simulink model "lab7_sin_triangle_generator_inverter"  (R2024b)
settings: Solver=VariableStepAuto  StartTime=0.0  StopTime=1  RelTol=1e-3
libraries: spsIdealSwitchLib x4, spsTriangleGeneratorLib x2, spsDCVoltageSourceLib x1, spsSeriesRLCBranchLib x1, spsVoltageMeasurementLib x1, sps_lib x1
settings Model: Creator=Admin  LastModifiedBy=pragy
settings DataIOCC: ReturnWorkspaceOutputs=off

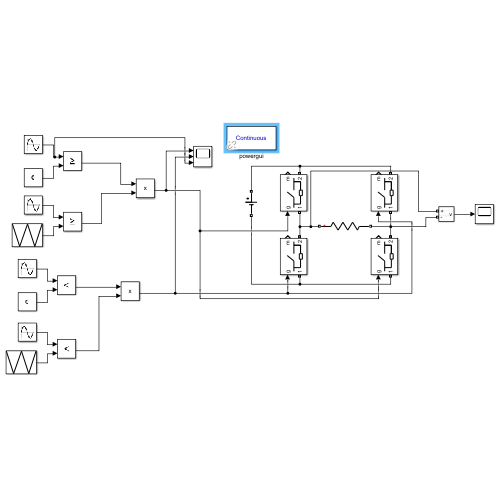
[thumbnail: Simulink's stored preview of the top-level diagram]
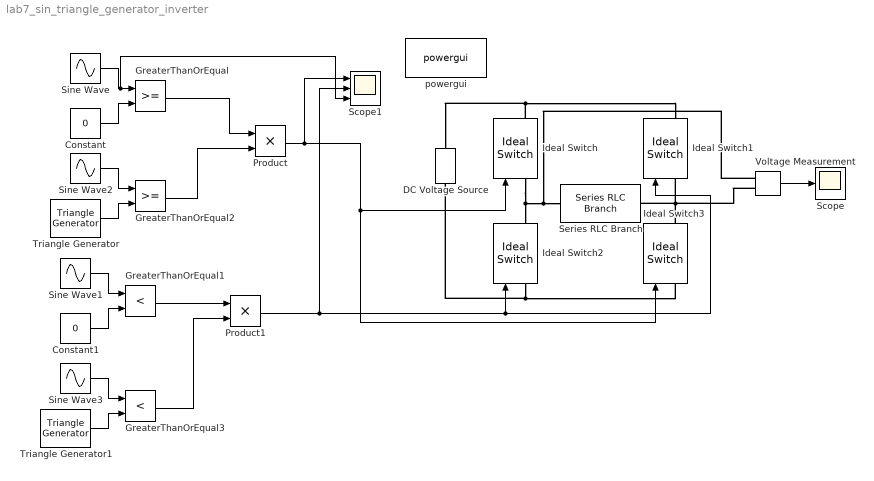
== system lab7_sin_triangle_generator_inverter ==
  Constant : Constant  Value=0
  Constant1 : Constant  Value=0
  DC Voltage Source : spsDCVoltageSourceLib/DC Voltage Source  Amplitude=220  Measurements=None
  GreaterThanOrEqual : RelationalOperator  OutDataTypeStr=boolean  RndMeth=Simplest  InputSameDT=off
  GreaterThanOrEqual1 : RelationalOperator  Operator=<  OutDataTypeStr=boolean  RndMeth=Simplest  InputSameDT=off
  GreaterThanOrEqual2 : RelationalOperator  OutDataTypeStr=boolean  RndMeth=Simplest  InputSameDT=off
  GreaterThanOrEqual3 : RelationalOperator  Operator=<  OutDataTypeStr=boolean  RndMeth=Simplest  InputSameDT=off
  Ideal Switch{,1..3} (4 alike) : spsIdealSwitchLib/Ideal Switch  Ron=0.001  Lon=0  IC=0  Rs=1e5  Cs=inf  Measurements=on
  Product : Product
  Product1 : Product
  Scope : Scope
  Scope1 : Scope  NumInputPorts=3
  Series RLC Branch : spsSeriesRLCBranchLib/Series RLC Branch  LConnTagsString=__new0  RConnTagsString=__new0  BranchType=R  Resistance=10  Inductance=1e-3  SetiL0=off  InitialCurrent=0  Capacitance=1e-6  Setx0=off  InitialVoltage=0  Measurements=None
  Sine Wave{,1..3} (4 alike) : Sin  Frequency=2*pi*50  SampleTime=0
  Triangle Generator : spsTriangleGeneratorLib/Triangle Generator  Freq=1050  Phase=180  Ts=0
  Triangle Generator1 : spsTriangleGeneratorLib/Triangle Generator  Freq=1050  Phase=180  Ts=0
  Voltage Measurement : spsVoltageMeasurementLib/Voltage Measurement  PhasorSimulation=off  OutputType=Complex  PSBequivalent=0
  powergui : sps_lib/powergui  Priority=1  SimulationMode=Continuous  SampleTime=50e-6  frequency=50  Iterations=50  frequencyindice=0  Pbase=100e6  ErrMax=1e-4  UnitsV=kV  UnitsW=MW  buscounter=0  FunctionMessages=off  echomessages=off  EnableUseOfTLC=off  CurrentSourceSwitches=off  DisableSnubberDevices=off  DisableRonSwitches=off  DisableVfSwitches=off  DisplayEquations=off  AutomaticDiscreteSolvers=off  SolverType=Tustin/Backward Euler (TBE)  Interpol=off  ExternalGateDelay=off  methode=off  Ts=100  x0status=zero  SPID=on  SwTol=0  HookPort=off  NonlinearTolerance=1e-4  nMaxIteration=100  ContinueOnMaxIteration=off  RestoreLinks=warning  ResistiveCurrentMeasurement=off  Frange=[0:2:500]  Ylog=off  Xlog=on  ShowGrid=off  save=off  variable=ZData  structure=0  ZoomFFT=off  StartTime=0.0  cycles=1  DisplayStyle=1  fundamental=60  FreqAxis=off  MaxFrequency=1000  frequencyindicesteady=1  RmsSteady=1  display=off
  wires:
  Constant/1 -> GreaterThanOrEqual/2
  GreaterThanOrEqual/1 -> Product/1
  Sine Wave/1 -> Scope1/3, GreaterThanOrEqual/1
  Constant1/1 -> GreaterThanOrEqual1/2
  Sine Wave1/1 -> GreaterThanOrEqual1/1
  GreaterThanOrEqual1/1 -> Product1/1
  Voltage Measurement/1 -> Scope/1
  Sine Wave2/1 -> GreaterThanOrEqual2/1
  Triangle Generator/1 -> GreaterThanOrEqual2/2
  Triangle Generator1/1 -> GreaterThanOrEqual3/2
  Sine Wave3/1 -> GreaterThanOrEqual3/1
  GreaterThanOrEqual2/1 -> Product/2
  GreaterThanOrEqual3/1 -> Product1/2
  Product/1 -> Ideal Switch3/1, Ideal Switch/1, Scope1/1
  Product1/1 -> Scope1/2, Ideal Switch1/1, Ideal Switch2/1
  connections:
  Ideal Switch/LConn1 -- Ideal Switch2/RConn1 -- Voltage Measurement/LConn1 -- Series RLC Branch/LConn1
  Ideal Switch3/RConn1 -- Series RLC Branch/RConn1 -- Voltage Measurement/LConn2 -- Ideal Switch1/LConn1
  Ideal Switch2/LConn1 -- DC Voltage Source/LConn1 -- Ideal Switch3/LConn1
  Ideal Switch/RConn1 -- DC Voltage Source/RConn1 -- Ideal Switch1/RConn1
